simulink model "project2Nonlinear"  (R2018b)
settings: Solver=FixedStepAuto  StartTime=0.0  StopTime=10.0  FixedStep=0.0005  RelTol=1e-3
settings Model: Creator=Young Wang  LastModifiedBy=Young Wang

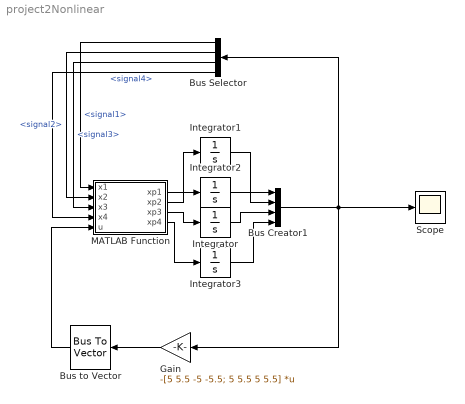
== system project2Nonlinear ==
  Bus Creator1 : BusCreator  Inputs=4
  Bus Selector : BusSelector  OutputSignals=signal1,signal2,signal3,signal4
  Bus to Vector : BusToVector
  Gain : Gain  Gain=-[5 5.5 -5 -5.5; 5 5.5 5 5.5]  Multiplication=Matrix(K*u)
  Integrator{,1..3} (4 alike) : Integrator  InitialCondition=1
  MATLAB Function : MATLAB Function  TreatAsAtomicUnit=on
  Scope : Scope
  wires:
  Gain/1 -> Bus to Vector/1
  Bus to Vector/1 -> MATLAB Function/5(u)
  Integrator2/1 -> Bus Creator1/1
  MATLAB Function/1(xp1) -> Integrator2/1
  Integrator1/1 -> Bus Creator1/2
  MATLAB Function/2(xp2) -> Integrator1/1
  Integrator3/1 -> Bus Creator1/4
  MATLAB Function/4(xp4) -> Integrator3/1
  Integrator/1 -> Bus Creator1/3
  MATLAB Function/3(xp3) -> Integrator/1
  Bus Creator1/1 -> Bus Selector/1, Gain/1, Scope/1
  Bus Selector/1 -> MATLAB Function/1(x1)  "<signal1>"
  Bus Selector/2 -> MATLAB Function/2(x2)  "<signal2>"
  Bus Selector/3 -> MATLAB Function/3(x3)  "<signal3>"
  Bus Selector/4 -> MATLAB Function/4(x4)  "<signal4>"

== matlab function project2Nonlinear/MATLAB Function ==
  data: x1 input; x2 input; x3 input; x4 input; u input; xp1 output; xp2 output; xp3 output; xp4 output
function [xp1, xp2, xp3, xp4] = fcn(x1,x2,x3,x4,u)
% constants
l = 0;
M = 0;
J = 0;
g = 9.81;
% states
% x1 = x(1);
% x2 = x(2);
% x3 = x(3);
% x4 = x(4);
% inputs
F1 = u(1);
F2 = u(2);
% nonlinear equations
xp1 = x2;
xp2 = ((F1+F2)/M)*cos(x3)+g;
xp3 = x4;
xp4 = ((F2-F2)/J)*l;
xp = [xp1; xp2; xp3; xp4];
y = xp;
